simulink model "LorenzAttractor"  (R2021b)
settings: Solver=VariableStepAuto  StartTime=0.0  StopTime=10  RelTol=1e-3
settings Model: Creator=anna  LastModifiedBy=anna

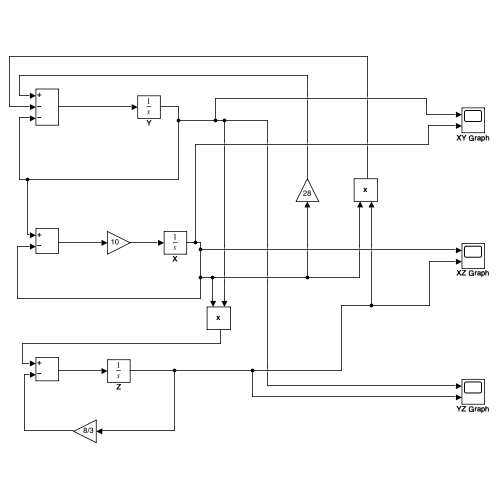
[thumbnail: Simulink's stored preview of the top-level diagram]
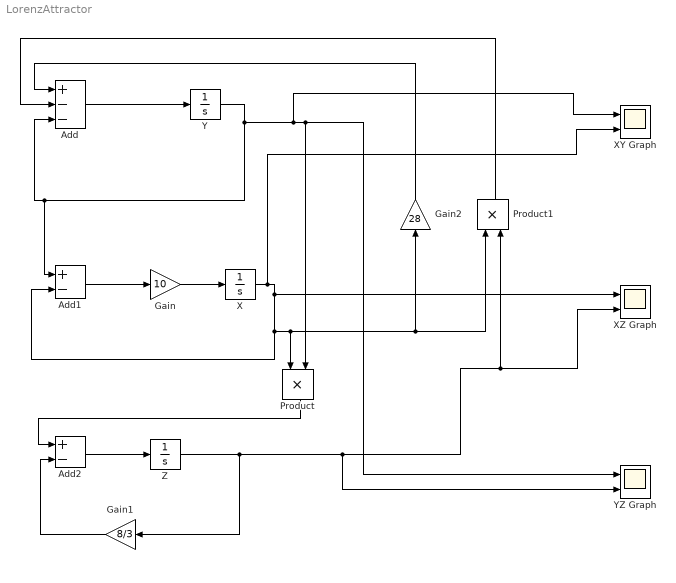
== system LorenzAttractor ==
  Add : Sum  Inputs=+--
  Add1 : Sum  Inputs=+-
  Add2 : Sum  Inputs=+-
  Gain : Gain  Gain=10
  Gain1 : Gain  Gain=8/3
  Gain2 : Gain  Gain=28
  Product : Product
  Product1 : Product
  X : Integrator  InitialCondition=2
  XY Graph : Scope  NumInputPorts=2
  XZ Graph : Scope  NumInputPorts=2
  Y : Integrator
  YZ Graph : Scope  NumInputPorts=2
  Z : Integrator  InitialCondition=20
  wires:
  Add/1 -> Y/1
  Gain2/1 -> Add/1
  Y/1 -> YZ Graph/1, Product/2, XY Graph/1, Add1/1, Add/3
  Add1/1 -> Gain/1
  Gain/1 -> X/1
  Product1/1 -> Add/2
  Product/1 -> Add2/1
  Gain1/1 -> Add2/2
  Add2/1 -> Z/1
  Z/1 -> Gain1/1, YZ Graph/2, XZ Graph/2, Product1/2
  X/1 -> XZ Graph/1, Product1/1, Gain2/1, Product/1, Add1/2, XY Graph/2
